simulink model "simulink_8bus"  (R2021b)
settings: Solver=VariableStepAuto  StartTime=0.0  StopTime=10.0  RelTol=1e-3
libraries: spsLoadFlowBusLib x9, spsThreePhasePISectionLineLib x8, spsThreePhaseParallelRLCLoadLib x7, spsThreePhaseSourceLib x1, spsThreePhaseTransformerTwoWindingsLib x1, spspowerguiLib x1
settings Model: Creator=xjk374  LastModifiedBy=Rey

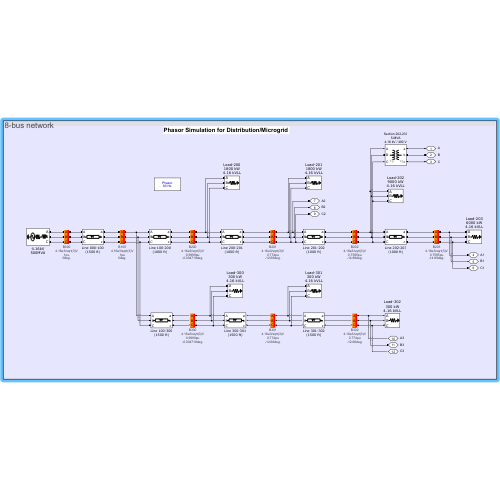
[thumbnail: Simulink's stored preview of the top-level diagram]
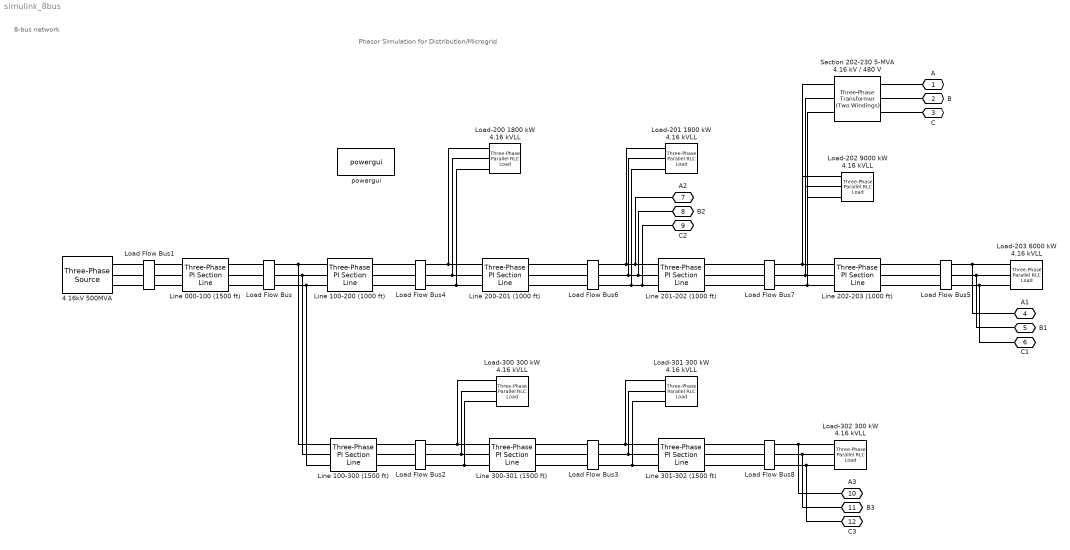
== system simulink_8bus ==
  note: 8-bus network
  note: Phasor Simulation for Distribution/Microgrid
  4.16kV 500MVA : spsThreePhaseSourceLib/Three-Phase Source  InternalConnection=Yg  VoltagePhases=on  Voltage=13e3  PhaseAngle=0  Voltage_phases=[ 1.012 1.0132 1.01247]*2401.8  PhaseAngles_phases=[ 2.72864 -117.277 122.694]  Frequency=60  NonIdealSource=on  SpecifyImpedance=on  Resistance=0.8929  Inductance=16.58e-3  ShortCircuitLevel=500e6  BaseVoltage=4.16e3  XRratio=16  BusType=swing  Pref=0  Qref=0  Prefabc=[0 0 0]  Qrefabc=[0 0 0]  Qmin=-inf  Qmax=inf
  Line 000-100 (1500 ft) : spsThreePhasePISectionLineLib/Three-Phase PI Section Line  LConnTagsString=a|b|c  RConnTagsString=A|B|C  Length=0.4572  Frequency=60  Resistances=[0.105 0.3558]  Inductances=[1.05e-3 3.32e-3]  Capacitances=[11.33e-009 5.01e-009]
  Line 100-200 (1000 ft) : spsThreePhasePISectionLineLib/Three-Phase PI Section Line  LConnTagsString=a|b|c  RConnTagsString=A|B|C  Length=0.3048  Frequency=60  Resistances=[0.105 0.3558]  Inductances=[1.05e-3 3.32e-3]  Capacitances=[11.33e-009 5.01e-009]
  Line 100-300 (1500 ft) : spsThreePhasePISectionLineLib/Three-Phase PI Section Line  LConnTagsString=a|b|c  RConnTagsString=A|B|C  Length=0.4572  Frequency=60  Resistances=[0.105 0.3558]  Inductances=[1.05e-3 3.32e-3]  Capacitances=[11.33e-009 5.01e-009]
  Line 200-201 (1000 ft) : spsThreePhasePISectionLineLib/Three-Phase PI Section Line  LConnTagsString=a|b|c  RConnTagsString=A|B|C  Length=0.3048  Frequency=60  Resistances=[0.105 0.3558]  Inductances=[1.05e-3 3.32e-3]  Capacitances=[11.33e-009 5.01e-009]
  Line 201-202 (1000 ft) : spsThreePhasePISectionLineLib/Three-Phase PI Section Line  LConnTagsString=a|b|c  RConnTagsString=A|B|C  Length=0.3048  Frequency=60  Resistances=[0.105 0.3558]  Inductances=[1.05e-3 3.32e-3]  Capacitances=[11.33e-009 5.01e-009]
  Line 202-203 (1000 ft) : spsThreePhasePISectionLineLib/Three-Phase PI Section Line  LConnTagsString=a|b|c  RConnTagsString=A|B|C  Length=0.3048  Frequency=60  Resistances=[0.105 0.3558]  Inductances=[1.05e-3 3.32e-3]  Capacitances=[11.33e-009 5.01e-009]
  Line 300-301 (1500 ft) : spsThreePhasePISectionLineLib/Three-Phase PI Section Line  LConnTagsString=a|b|c  RConnTagsString=A|B|C  Length=0.4572  Frequency=60  Resistances=[0.105 0.3558]  Inductances=[1.05e-3 3.32e-3]  Capacitances=[11.33e-009 5.01e-009]
  Line 301-302 (1500 ft) : spsThreePhasePISectionLineLib/Three-Phase PI Section Line  LConnTagsString=a|b|c  RConnTagsString=A|B|C  Length=0.4572  Frequency=60  Resistances=[0.105 0.3558]  Inductances=[1.05e-3 3.32e-3]  Capacitances=[11.33e-009 5.01e-009]
  Load Flow Bus : spsLoadFlowBusLib/Load Flow Bus  LConnTagsString=a|b|c  RConnTagsString=a|b|c  Phases=ABC  Connectors=on both sides  ID=B100  Vbase=4.16e3/sqrt(3)  Vref=[1.0 1.0 1.0]  Vangle=[0 -120 120]  VLF=1  VLFb=1  VLFc=1  angleLF=0  angleLFb=-120  angleLFc=120
      settings: SourceProductBaseCode=PS
  Load Flow Bus1 : spsLoadFlowBusLib/Load Flow Bus  LConnTagsString=a|b|c  RConnTagsString=a|b|c  Phases=ABC  Connectors=on both sides  ID=B000  Vbase=4.16e3/sqrt(3)  Vref=[1.0 1.0 1.0]  Vangle=[0 -120 120]  VLF=1  VLFb=1  VLFc=1  angleLF=0  angleLFb=-120  angleLFc=120
      settings: SourceProductBaseCode=PS
  Load Flow Bus2 : spsLoadFlowBusLib/Load Flow Bus  LConnTagsString=a|b|c  RConnTagsString=a|b|c  Phases=ABC  Connectors=on both sides  ID=B300  Vbase=4.16e3/sqrt(3)  Vref=[1.0 1.0 1.0]  Vangle=[0 -120 120]  VLF=0.9999  VLFb=0.9999  VLFc=0.9999  angleLF=-0.004718  angleLFb=-120  angleLFc=120
      settings: SourceProductBaseCode=PS
  Load Flow Bus3 : spsLoadFlowBusLib/Load Flow Bus  LConnTagsString=a|b|c  RConnTagsString=a|b|c  Phases=ABC  Connectors=on both sides  ID=B301  Vbase=4.16e3/sqrt(3)  Vref=[1.0 1.0 1.0]  Vangle=[0 -120 120]  VLF=0.774  VLFb=0.8072  VLFc=0.7635  angleLF=-12.66  angleLFb=-136.4  angleLFc=104.5
      settings: SourceProductBaseCode=PS
  Load Flow Bus4 : spsLoadFlowBusLib/Load Flow Bus  LConnTagsString=a|b|c  RConnTagsString=a|b|c  Phases=ABC  Connectors=on both sides  ID=B200  Vbase=4.16e3/sqrt(3)  Vref=[1.0 1.0 1.0]  Vangle=[0 -120 120]  VLF=0.9999  VLFb=0.9999  VLFc=0.9999  angleLF=-0.004718  angleLFb=-120  angleLFc=120
      settings: SourceProductBaseCode=PS
  Load Flow Bus5 : spsLoadFlowBusLib/Load Flow Bus  LConnTagsString=a|b|c  RConnTagsString=a|b|c  Phases=ABC  Connectors=on both sides  ID=B203  Vbase=4.16e3/sqrt(3)  Vref=[1.0 1.0 1.0]  Vangle=[0 -120 120]  VLF=0.7595  VLFb=0.8002  VLFc=0.7507  angleLF=-14.89  angleLFb=-138.9  angleLFc=101.8
      settings: SourceProductBaseCode=PS
  Load Flow Bus6 : spsLoadFlowBusLib/Load Flow Bus  LConnTagsString=a|b|c  RConnTagsString=a|b|c  Phases=ABC  Connectors=on both sides  ID=B201  Vbase=4.16e3/sqrt(3)  Vref=[1.0 1.0 1.0]  Vangle=[0 -120 120]  VLF=0.774  VLFb=0.8072  VLFc=0.7635  angleLF=-12.66  angleLFb=-136.4  angleLFc=104.5
      settings: SourceProductBaseCode=PS
  Load Flow Bus7 : spsLoadFlowBusLib/Load Flow Bus  LConnTagsString=a|b|c  RConnTagsString=a|b|c  Phases=ABC  Connectors=on both sides  ID=B202  Vbase=4.16e3/sqrt(3)  Vref=[1.0 1.0 1.0]  Vangle=[0 -120 120]  VLF=0.7595  VLFb=0.8002  VLFc=0.7507  angleLF=-14.89  angleLFb=-138.9  angleLFc=101.8
      settings: SourceProductBaseCode=PS
  Load Flow Bus8 : spsLoadFlowBusLib/Load Flow Bus  LConnTagsString=a|b|c  RConnTagsString=a|b|c  Phases=ABC  Connectors=on both sides  ID=B302  Vbase=4.16e3/sqrt(3)  Vref=[1.0 1.0 1.0]  Vangle=[0 -120 120]  VLF=0.774  VLFb=0.8072  VLFc=0.7635  angleLF=-12.66  angleLFb=-136.4  angleLFc=104.5
      settings: SourceProductBaseCode=PS
  Load-200 1800 kW 4.16 kVLL : spsThreePhaseParallelRLCLoadLib/Three-Phase Parallel RLC Load  LConnTagsString=A|B|C  Configuration=Y (grounded)  NominalVoltage=4160  Vabc=[1e3 1e3 1e3]  Vabcp=[1e3 1e3 1e3]  NominalFrequency=60  UnbalancedPower=off  ActivePower=1800e3  InductivePower=0  CapacitivePower=0  Pabc=[10e3 9e3 11e3]  QLabc=[100 90 110]  QCabc=[100 90 110]  Pabcp=[10e3 9e3 11e3]  QLabcp=[100 90 110]  QCabcp=[100 90 110]  Measurements=None  LoadType=constant PQ
  Load-201 1800 kW 4.16 kVLL : spsThreePhaseParallelRLCLoadLib/Three-Phase Parallel RLC Load  LConnTagsString=A|B|C  Configuration=Y (grounded)  NominalVoltage=4160  Vabc=[1e3 1e3 1e3]  Vabcp=[1e3 1e3 1e3]  NominalFrequency=60  UnbalancedPower=off  ActivePower=1800e3  InductivePower=0  CapacitivePower=0  Pabc=[10e3 9e3 11e3]  QLabc=[100 90 110]  QCabc=[100 90 110]  Pabcp=[10e3 9e3 11e3]  QLabcp=[100 90 110]  QCabcp=[100 90 110]  Measurements=None  LoadType=constant PQ
  Load-202 9000 kW 4.16 kVLL : spsThreePhaseParallelRLCLoadLib/Three-Phase Parallel RLC Load  LConnTagsString=A|B|C  Configuration=Y (grounded)  NominalVoltage=4160  Vabc=[1e3 1e3 1e3]  Vabcp=[1e3 1e3 1e3]  NominalFrequency=60  UnbalancedPower=off  ActivePower=9000e3  InductivePower=0  CapacitivePower=0  Pabc=[10e3 9e3 11e3]  QLabc=[100 90 110]  QCabc=[100 90 110]  Pabcp=[10e3 9e3 11e3]  QLabcp=[100 90 110]  QCabcp=[100 90 110]  Measurements=None  LoadType=constant PQ
  Load-203 6000 kW 4.16 kVLL : spsThreePhaseParallelRLCLoadLib/Three-Phase Parallel RLC Load  LConnTagsString=A|B|C  Configuration=Y (grounded)  NominalVoltage=4160  Vabc=[1e3 1e3 1e3]  Vabcp=[1e3 1e3 1e3]  NominalFrequency=60  UnbalancedPower=off  ActivePower=6000e-3  InductivePower=0  CapacitivePower=0  Pabc=[10e3 9e3 11e3]  QLabc=[100 90 110]  QCabc=[100 90 110]  Pabcp=[10e3 9e3 11e3]  QLabcp=[100 90 110]  QCabcp=[100 90 110]  Measurements=None  LoadType=constant PQ
  Load-300 300 kW 4.16 kVLL : spsThreePhaseParallelRLCLoadLib/Three-Phase Parallel RLC Load  LConnTagsString=A|B|C  Configuration=Y (grounded)  NominalVoltage=4160  Vabc=[1e3 1e3 1e3]  Vabcp=[1e3 1e3 1e3]  NominalFrequency=60  UnbalancedPower=off  ActivePower=300e3  InductivePower=0  CapacitivePower=0  Pabc=[10e3 9e3 11e3]  QLabc=[100 90 110]  QCabc=[100 90 110]  Pabcp=[10e3 9e3 11e3]  QLabcp=[100 90 110]  QCabcp=[100 90 110]  Measurements=None  LoadType=constant PQ
  Load-301 300 kW 4.16 kVLL : spsThreePhaseParallelRLCLoadLib/Three-Phase Parallel RLC Load  LConnTagsString=A|B|C  Configuration=Y (grounded)  NominalVoltage=4160  Vabc=[1e3 1e3 1e3]  Vabcp=[1e3 1e3 1e3]  NominalFrequency=60  UnbalancedPower=off  ActivePower=300e3  InductivePower=0  CapacitivePower=0  Pabc=[10e3 9e3 11e3]  QLabc=[100 90 110]  QCabc=[100 90 110]  Pabcp=[10e3 9e3 11e3]  QLabcp=[100 90 110]  QCabcp=[100 90 110]  Measurements=None  LoadType=constant PQ
  Load-302 300 kW 4.16 kVLL : spsThreePhaseParallelRLCLoadLib/Three-Phase Parallel RLC Load  LConnTagsString=A|B|C  Configuration=Y (grounded)  NominalVoltage=4160  Vabc=[1e3 1e3 1e3]  Vabcp=[1e3 1e3 1e3]  NominalFrequency=60  UnbalancedPower=off  ActivePower=300e-3  InductivePower=0  CapacitivePower=0  Pabc=[10e3 9e3 11e3]  QLabc=[100 90 110]  QCabc=[100 90 110]  Pabcp=[10e3 9e3 11e3]  QLabcp=[100 90 110]  QCabcp=[100 90 110]  Measurements=None  LoadType=constant PQ
  Section 202-230 5-MVA 4.16 kV / 480 V : spsThreePhaseTransformerTwoWindingsLib/Three-Phase Transformer (Two Windings)  Winding1Connection=Yg  Winding2Connection=Yg  CoreType=Three single-phase transformers  SetSaturation=off  Hysteresis=off  DataFile='hysteresis'  SetInitialFlux=off  Measurements=None  UNITS=pu  NominalPower=[5e6 , 60 ]  Winding1=[ 4.16e3 , 0.01 , 0.088 ]  Winding2=[480 , 0.001 , 0.001 ]  Rm=500  Lm=500  L0=0.5  Saturation=[ 0,0 ; 0.0024,1.2 ; 1.0,1.52 ]  InitialFluxes=[ 0.8 , -0.8 , 0.7 ]  BreakLoop=off  DiscreteSolver=Trapezoidal iterative  DataType=off  TransfoNumber=0
  powergui : spspowerguiLib/powergui  Priority=1  SimulationMode=Phasor  SampleTime=50e-6  frequency=60  Iterations=50  frequencyindice=60  Pbase=100e6  ErrMax=1e-4  UnitsV=kV  UnitsW=MW  buscounter=0  FunctionMessages=off  echomessages=off  EnableUseOfTLC=off  CurrentSourceSwitches=off  DisableSnubberDevices=off  DisableRonSwitches=off  DisableVfSwitches=off  DisplayEquations=off  AutomaticDiscreteSolvers=off  SolverType=Tustin/Backward Euler (TBE)  Interpol=off  ExternalGateDelay=off  methode=off  Ts=100  x0status=blocks  SPID=on  SwTol=0  HookPort=off  NonlinearTolerance=1e-4  nMaxIteration=100  ContinueOnMaxIteration=off  RestoreLinks=warning  ResistiveCurrentMeasurement=off  Frange=[0:2:500]  Ylog=off  Xlog=on  ShowGrid=off  save=off  variable=ZData  structure=0  ZoomFFT=off  StartTime=0.0  cycles=1  DisplayStyle=1  fundamental=60  FreqAxis=off  MaxFrequency=1000  frequencyindicesteady=1  RmsSteady=1  display=off
  A : PMIOPort  Side=Left
  B : PMIOPort  Port=2  Side=Left
  C : PMIOPort  Port=3  Side=Left
  A1 : PMIOPort  Port=4  Side=Left
  B1 : PMIOPort  Port=5  Side=Left
  C1 : PMIOPort  Port=6  Side=Left
  A2 : PMIOPort  Port=7  Side=Left
  B2 : PMIOPort  Port=8  Side=Left
  C2 : PMIOPort  Port=9  Side=Left
  A3 : PMIOPort  Port=10  Side=Left
  B3 : PMIOPort  Port=11  Side=Left
  C3 : PMIOPort  Port=12  Side=Left
  connections:
  Line 201-202 (1000 ft)/RConn3 -- Load Flow Bus7/LConn3
  Line 201-202 (1000 ft)/RConn1 -- Load Flow Bus7/LConn1
  Line 201-202 (1000 ft)/RConn2 -- Load Flow Bus7/LConn2
  Load-201 1800 kW 4.16 kVLL/LConn1 -- Load Flow Bus6/RConn1 -- A2/RConn1 -- Line 201-202 (1000 ft)/LConn1
  Line 200-201 (1000 ft)/LConn2 -- Load-200 1800 kW 4.16 kVLL/LConn2 -- Load Flow Bus4/RConn2
  Line 200-201 (1000 ft)/RConn3 -- Load Flow Bus6/LConn3
  Line 000-100 (1500 ft)/RConn1 -- Load Flow Bus/LConn1
  Section 202-230 5-MVA 4.16 kV / 480 V/RConn2 -- B/RConn1
  Section 202-230 5-MVA 4.16 kV / 480 V/RConn3 -- C/RConn1
  Line 100-200 (1000 ft)/RConn3 -- Load Flow Bus4/LConn3
  Section 202-230 5-MVA 4.16 kV / 480 V/RConn1 -- A/RConn1
  Line 200-201 (1000 ft)/LConn1 -- Load-200 1800 kW 4.16 kVLL/LConn1 -- Load Flow Bus4/RConn1
  Line 200-201 (1000 ft)/RConn1 -- Load Flow Bus6/LConn1
  Line 100-200 (1000 ft)/RConn2 -- Load Flow Bus4/LConn2
  Line 200-201 (1000 ft)/LConn3 -- Load Flow Bus4/RConn3 -- Load-200 1800 kW 4.16 kVLL/LConn3
  Line 000-100 (1500 ft)/RConn2 -- Load Flow Bus/LConn2
  Line 100-200 (1000 ft)/LConn2 -- Load Flow Bus/RConn2 -- Line 100-300 (1500 ft)/LConn2
  Line 100-200 (1000 ft)/LConn1 -- Load Flow Bus/RConn1 -- Line 100-300 (1500 ft)/LConn1
  Line 100-200 (1000 ft)/LConn3 -- Load Flow Bus/RConn3 -- Line 100-300 (1500 ft)/LConn3
  Line 100-200 (1000 ft)/RConn1 -- Load Flow Bus4/LConn1
  Line 000-100 (1500 ft)/RConn3 -- Load Flow Bus/LConn3
  Line 200-201 (1000 ft)/RConn2 -- Load Flow Bus6/LConn2
  Load Flow Bus1/LConn1 -- 4.16kV 500MVA/RConn1
  Load Flow Bus1/LConn2 -- 4.16kV 500MVA/RConn2
  Load Flow Bus1/LConn3 -- 4.16kV 500MVA/RConn3
  Load Flow Bus1/RConn1 -- Line 000-100 (1500 ft)/LConn1
  Load Flow Bus1/RConn2 -- Line 000-100 (1500 ft)/LConn2
  Load Flow Bus1/RConn3 -- Line 000-100 (1500 ft)/LConn3
  Load Flow Bus2/LConn1 -- Line 100-300 (1500 ft)/RConn1
  Load Flow Bus2/LConn2 -- Line 100-300 (1500 ft)/RConn2
  Load Flow Bus2/LConn3 -- Line 100-300 (1500 ft)/RConn3
  Line 300-301 (1500 ft)/LConn1 -- Load-300 300 kW 4.16 kVLL/LConn1 -- Load Flow Bus2/RConn1
  Line 300-301 (1500 ft)/LConn2 -- Load-300 300 kW 4.16 kVLL/LConn2 -- Load Flow Bus2/RConn2
  Line 300-301 (1500 ft)/LConn3 -- Load-300 300 kW 4.16 kVLL/LConn3 -- Load Flow Bus2/RConn3
  Load Flow Bus3/LConn2 -- Line 300-301 (1500 ft)/RConn2
  Load Flow Bus3/LConn1 -- Line 300-301 (1500 ft)/RConn1
  Load Flow Bus3/LConn3 -- Line 300-301 (1500 ft)/RConn3
  Line 301-302 (1500 ft)/LConn1 -- Load-301 300 kW 4.16 kVLL/LConn1 -- Load Flow Bus3/RConn1
  Line 301-302 (1500 ft)/LConn2 -- Load-301 300 kW 4.16 kVLL/LConn2 -- Load Flow Bus3/RConn2
  Line 301-302 (1500 ft)/LConn3 -- Load-301 300 kW 4.16 kVLL/LConn3 -- Load Flow Bus3/RConn3
  Load-203 6000 kW 4.16 kVLL/LConn1 -- A1/RConn1 -- Load Flow Bus5/RConn1
  Load-203 6000 kW 4.16 kVLL/LConn2 -- B1/RConn1 -- Load Flow Bus5/RConn2
  Load-203 6000 kW 4.16 kVLL/LConn3 -- C1/RConn1 -- Load Flow Bus5/RConn3
  Line 202-203 (1000 ft)/LConn1 -- Section 202-230 5-MVA 4.16 kV / 480 V/LConn1 -- Load-202 9000 kW 4.16 kVLL/LConn1 -- Load Flow Bus7/RConn1
  Line 202-203 (1000 ft)/LConn2 -- Section 202-230 5-MVA 4.16 kV / 480 V/LConn2 -- Load-202 9000 kW 4.16 kVLL/LConn2 -- Load Flow Bus7/RConn2
  Line 202-203 (1000 ft)/LConn3 -- Section 202-230 5-MVA 4.16 kV / 480 V/LConn3 -- Load-202 9000 kW 4.16 kVLL/LConn3 -- Load Flow Bus7/RConn3
  Line 202-203 (1000 ft)/RConn1 -- Load Flow Bus5/LConn1
  Line 202-203 (1000 ft)/RConn2 -- Load Flow Bus5/LConn2
  Line 202-203 (1000 ft)/RConn3 -- Load Flow Bus5/LConn3
  Load Flow Bus8/LConn1 -- Line 301-302 (1500 ft)/RConn1
  Load Flow Bus8/LConn2 -- Line 301-302 (1500 ft)/RConn2
  Load Flow Bus8/LConn3 -- Line 301-302 (1500 ft)/RConn3
  Load-302 300 kW 4.16 kVLL/LConn1 -- A3/RConn1 -- Load Flow Bus8/RConn1
  Load-302 300 kW 4.16 kVLL/LConn2 -- B3/RConn1 -- Load Flow Bus8/RConn2
  Load-302 300 kW 4.16 kVLL/LConn3 -- C3/RConn1 -- Load Flow Bus8/RConn3
  Load Flow Bus6/RConn2 -- Load-201 1800 kW 4.16 kVLL/LConn2 -- B2/RConn1 -- Line 201-202 (1000 ft)/LConn2
  Load Flow Bus6/RConn3 -- Load-201 1800 kW 4.16 kVLL/LConn3 -- C2/RConn1 -- Line 201-202 (1000 ft)/LConn3
